simulink model "baleka2S_simscape_frame"  (R2024b)
settings: Solver=VariableStepAuto  StartTime=0.0  StopTime=7.5  RelTol=1e-3
InitFcn:
  | VLcmdsignal = struct( ...
  |     'r_des', 0.45, ...
  |     'dr_des', 0, ...
  |     'th_des', -pi/2, ...
  |     'dth_des', 0, ...
  |     'KPr', 200, ...
  |     'KDr', 2, ...
  |     'KPth', 30, ...
  |     'KDth', 4, ...
  |     'Fff', 0, ...
  |     'Tff', 0);
  | 
  | % run("roll_body_DataFile.m");
  | % run("diff_body_DataFile.m");
undefined symbols (not defined in the file): Kd, Kp, q, tff, w, X, Y, Z
libraries: sm_lib x123, nesl_utility x13, aru_toolbox x11
(part 1 of 3)
settings Model: DataDictionary=Library_dictionary.sldd  Creator=claro  LastModifiedBy=claro

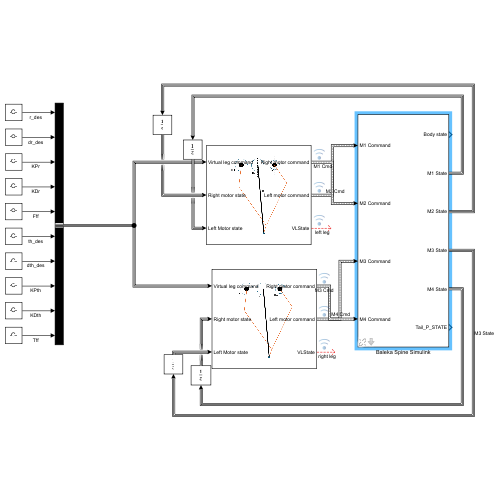
[thumbnail: Simulink's stored preview of the top-level diagram]
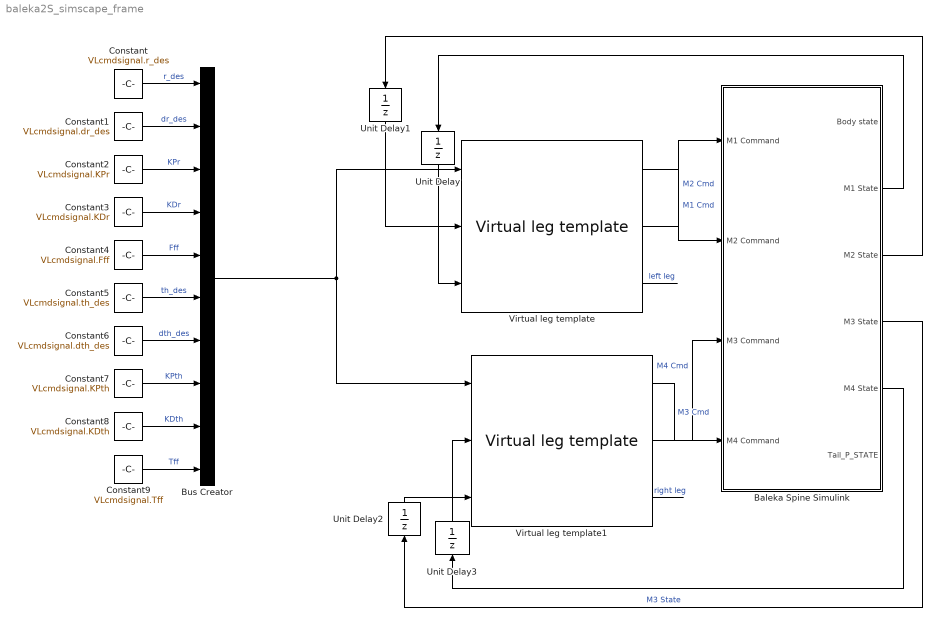
== system baleka2S_simscape_frame ==
  Baleka Spine Simulink : Subsystem  AncestorBlock=aru_toolbox/Baleka 2.5/Baleka Simscape  mask(Simulation model){communication_rate=1000, GravityBool=on, mu_s=1, mu_k=0.9, foot_k=1e5, foot_d=1e4, y_start=0.35, StartingMode=Zero (set Starting values manually), LOffset=2*pi-2.7, ROffset=-0.3}
      mask prompts: communication_rate "Communication Rate"; GravityBool "Enable gravity"; mu_s "Static friction coefficient"; mu_k "Kinetic Friction coefficient"; foot_k "Contact spring constant"; foot_d "Contact damping"; y_start "Boom height (m)"; StartingMode "Starting angle preset"; LOffset "Left motor starting angles (rad)"; ROffset "Right motor starting angles (rad)"
      mask help: The (hopefully) all-in-one model for simulating Baleka 2.5 using Simscape. This model assumes counter clockwise positive, and has busses for both inputs and outputs.
      mask init:
      | if StartingMode == "Crouched"
      |         LmotorOffset = pi-37.63*pi/180; % Measured from Solidworks model and confirmed in Simscape
      |         RmotorOffset = 38.24*pi/180;
      |         LinkStartingRad=1;
      |         
      |     end
      |     if StartingMode == "Links horizontal"
      |         LmotorOffset = pi;
      |         RmotorOffset =0;
      |         LinkStartingRad = 2;
      |     end
      |     if StartingMode == "Zero (set Starting values manually)"
      |         LmotorOffset = LOffset;
      |         RmotorOffset = ROffset;
      |         LinkStartingRad=0;
      |     end
      |    if GravityBool
      |        g = -9.80665;
      |    else
      |        g = 0;
      |    end
      |    th_boom = asin((y_start -0.101)/2.493);
      mask TypeOptions StartingMode: Crouched | Links horizontal | Zero (set Starting values manually)
      mask DialogControl Container3 Prompt: Contacts
      mask DialogControl Container4 Prompt: Starting values
      mask DialogControl Container5 Prompt: Leg angles
      mask DialogControl Control2 Prompt: Custom angles only implimented if starting preset is zero
  Bus Creator : BusCreator  Inputs=10  OutDataTypeStr=Bus: VLcmd
  Constant : Constant  Value=VLcmdsignal.r_des
  Constant1 : Constant  Value=VLcmdsignal.dr_des
  Constant2 : Constant  Value=VLcmdsignal.KPr
  Constant3 : Constant  Value=VLcmdsignal.KDr
  Constant4 : Constant  Value=VLcmdsignal.Fff
  Constant5 : Constant  Value=VLcmdsignal.th_des
  Constant6 : Constant  Value=VLcmdsignal.dth_des
  Constant7 : Constant  Value=VLcmdsignal.KPth
  Constant8 : Constant  Value=VLcmdsignal.KDth
  Constant9 : Constant  Value=VLcmdsignal.Tff
  Unit Delay{,1..3} (4 alike) : UnitDelay  SampleTime=-1  HasFrameUpgradeWarning=on
  Virtual leg template : aru_toolbox/Baleka 2.5/Virtual leg template  SystemSampleTime=-1  VariantActivationTime=update diagram  AllowFlexibleInterface=on  Latency=0  AutoFrameSizeCalculation=off
      settings: SourceProductName=ARU Toolbox
  Virtual leg template1 : aru_toolbox/Baleka 2.5/Virtual leg template  SystemSampleTime=-1  VariantActivationTime=update diagram  AllowFlexibleInterface=on  Latency=0  AutoFrameSizeCalculation=off
      settings: SourceProductName=ARU Toolbox
  wires:
  Virtual leg template/2 -> Baleka Spine Simulink/1(M1 Command)  "M2 Cmd"
  Virtual leg template/1 -> Baleka Spine Simulink/2(M2 Command)  "M1 Cmd"
  Virtual leg template1/1 -> Baleka Spine Simulink/4(M4 Command)  "M3 Cmd"
  Virtual leg template1/2 -> Baleka Spine Simulink/3(M3 Command)  "M4 Cmd"
  Baleka Spine Simulink/4(M3 State) -> Unit Delay2/1  "M3 State"
  Bus Creator/1 -> Virtual leg template/1, Virtual leg template1/1
  Constant/1 -> Bus Creator/1  "r_des"
  Constant1/1 -> Bus Creator/2  "dr_des"
  Constant2/1 -> Bus Creator/3  "KPr"
  Constant3/1 -> Bus Creator/4  "KDr"
  Constant4/1 -> Bus Creator/5  "Fff"
  Constant5/1 -> Bus Creator/6  "th_des"
  Constant6/1 -> Bus Creator/7  "dth_des"
  Constant7/1 -> Bus Creator/8  "KPth"
  Constant8/1 -> Bus Creator/9  "KDth"
  Constant9/1 -> Bus Creator/10  "Tff"
  Unit Delay/1 -> Virtual leg template/3
  Unit Delay1/1 -> Virtual leg template/2
  Unit Delay2/1 -> Virtual leg template1/3
  Unit Delay3/1 -> Virtual leg template1/2
  Baleka Spine Simulink/5(M4 State) -> Unit Delay3/1
  Baleka Spine Simulink/2(M1 State) -> Unit Delay/1
  Baleka Spine Simulink/3(M2 State) -> Unit Delay1/1
  Virtual leg template1/3 -> ?  "right leg"
  Virtual leg template/3 -> ?  "left leg"

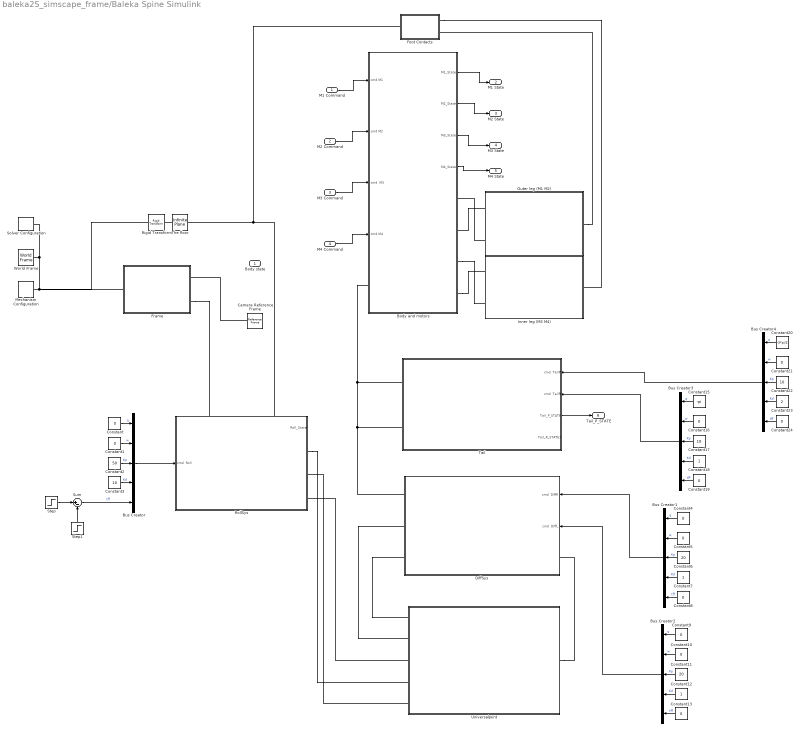
== system baleka2S_simscape_frame/Baleka Spine Simulink ==
  M1 Command : Inport  OutDataTypeStr=Bus: MotorCmd
  M2 Command : Inport  Port=2  OutDataTypeStr=Bus: MotorCmd
  M3 Command : Inport  Port=3  OutDataTypeStr=Bus: MotorCmd
  M4 Command : Inport  Port=4  OutDataTypeStr=Bus: MotorCmd
  " Outer leg (M1 M2)" : Subsystem
  Body and motors : Subsystem
  Bus Creator{,1..4} (5 alike) : BusCreator  Inputs=q,w,Kp,Kd,tff  OutDataTypeStr=Bus: MotorCmd
  Camera Reference Frame : sm_lib/Frames and Transforms/Reference Frame
  Constant{,1,4..5,8..10,13,16,19,21,24} (12 alike) : Constant  Value=0
  Constant11 : Constant  Value=20
  Constant12 : Constant
  Constant15 : Constant  Value=-pi
  Constant17 : Constant  Value=10
  Constant18 : Constant
  Constant2 : Constant  Value=50
  Constant20 : Constant  Value=-3*pi/2
  Constant22 : Constant  Value=10
  Constant23 : Constant  Value=2
  Constant3 : Constant  Value=10
  Constant6 : Constant  Value=20
  Constant7 : Constant
  DiffSys : Subsystem
      settings: PortSchema="{\"entries\":[{\"content\":{\"sides\":[{\"content\":{\"connectorIds\":[\"LConn1\",\"LConn2\",\"LConn3\"]},\"type\":\"ConnectorPlacement.EquallySpacedRectSide\",\"uuid\":\"322efe47-c693-4372-b523-ac4150ea56a3\"},{\"content\":{\"connectorIds\":[\"In1\",\"In2\",\"RConn1\"],\"side\":\"RIGHT\"},\"type\":\"ConnectorPlacement.EquallySpacedRectSide\",\"uuid\":\"9b382245-60e0-481a-af9a-4690adad6086\"},{\"content\":{\"side\":\"TOP\"},\"type\":\"ConnectorPlacement.EquallySpacedRectSide\",\"uuid\":\"0b256e53-2003-47ff-95d4-d002f32bb36d\"},{\"content\":{\"side\":\"BOTTOM\"},\"type\":\"ConnectorPlacement.EquallySpacedRectSide\",\"uuid\":\"ab3905eb-9bc7-48cc-903a-2471c31a1ad7\"}]},\"type\":\"ConnectorPlacement.EquallySpacedConnector\",\"uuid\":\"7ff5e8a9-a8e4-454d-a7ba-3a225b667645\"}],\"packageUris\":[\"http://schema.mathworks.com/mf0/Connector/R2020b\"],\"version\":\"1.0\"}"
  Foot Contacts : Subsystem
  Frame : Subsystem
  Inner leg (M3 M4) : Subsystem
  Mechanism Configuration : sm_lib/Utilities/Mechanism Configuration  UniformGravity=Constant  GravityVector=[0 0 g]  GravityVectorUnits=m/s^2  LinearizationDelta=0.001  JointModeTransitionNonlinearIterations=2
  Rigid Transform : sm_lib/Frames and Transforms/Rigid Transform  RotationMethod=None  FollAlignAxisA=+X  BaseAlignAxisA=+Y  FollAlignAxisB=+Y  BaseAlignAxisB=+Z  RotationStandardAxis=+Z  RotationAngle=0  RotationAngleUnits=deg  RotationArbitraryAxis=[0 0 1]  RotationSequenceAxes=FollowerAxes  RotationSequence=XYX  RotationSequenceAngles=[0 0 0]  RotationSequenceAnglesUnits=deg  RotationMatrix=[1 0 0;0 1 0;0 0 1]  Quaternion=[1 0 0 0]  TranslationMethod=Cartesian  TranslationCartesianOffset=[0 0 4]  TranslationCartesianOffsetUnits=mm  TranslationStandardAxis=+Z  TranslationStandardOffset=0  TranslationStandardOffsetUnits=m  TranslationROffset=0  TranslationROffsetUnits=m  TranslationThetaOffset=0  TranslationThetaOffsetUnits=deg  TranslationZOffset=0  TranslationZOffsetUnits=m
  RollSys : Subsystem
      settings: PortSchema="{\"entries\":[{\"content\":{\"sides\":[{\"content\":{\"connectorIds\":[\"In1\"]},\"type\":\"ConnectorPlacement.EquallySpacedRectSide\",\"uuid\":\"dfefdc23-044e-4fd3-8804-6b125fee8169\"},{\"content\":{\"connectorIds\":[\"Out1\",\"RConn1\",\"RConn2\",\"RConn3\"],\"side\":\"RIGHT\"},\"type\":\"ConnectorPlacement.EquallySpacedRectSide\",\"uuid\":\"fa13e48c-80ad-4683-8483-cd805fea927b\"},{\"content\":{\"connectorIds\":[\"LConn1\",\"LConn2\"],\"side\":\"TOP\"},\"type\":\"ConnectorPlacement.EquallySpacedRectSide\",\"uuid\":\"92ac139b-ee3c-4e16-9e24-f9ffaf9597bb\"}]},\"type\":\"ConnectorPlacement.EquallySpacedConnector\",\"uuid\":\"7d988bd9-98fd-44d8-87f5-37b6f9d1dfc6\"}],\"packageUris\":[\"http://schema.mathworks.com/mf0/Connector/R2020b\"],\"version\":\"1.0\"}"
  Solver Configuration : nesl_utility/Solver Configuration  PhysicalDomain=network_engine_domain  SubClassName=solver  LeftPortType=input  RightPortType=generic  Tones=[]  Harmonics=[]  SimulateNoise=off  Profile=off  UseLocalSampling=off  EnableSwitchedLinearOptims=on  FrequencyDomain=off  UseCCode=off  RelTol=0.001  AbsTol=1e-06  MinStep=1e-09  ToWorkspace=off  RevertToSquareIcSolve=off  NumHomotopyIterations=100  PhasorMode=off  PhasorModeNumHarmonics=1  ConsistencySolver=NEWTON_FTOL  IndexReductionMethod=DerivativeReplacement  DoDC=off  ResidualTolerance=1e-09  ConsistencyTolSource=GLOBAL  ConsistencyAbsTol=0.001  ConsistencyRelTol=0.001  ConsistencyTolFactor=0.001  UseLocalSolver=off  LocalSolverChoice=NE_BACKWARD_EULER_ADVANCER  ResolveIndetEquations=on  FunctionEvalNumThread=1  LocalSolverSampleTime=0.001  DoFixedCost=off  MaxNonlinIter=3  MaxModeIter=2  ComputeImpulses=off  ImpulseIterations=2  LinearAlgebra=Sparse  LinearAlgebraNumThread=0  EquationFormulation=NE_TIME_EF  DelaysMemoryBudget=1024  AutomaticFiltering=on  FilteringTimeConstant=0.001  PartitionStorageMethod=AS_NEEDED  PartitionMemoryBudget=1024  PartitionMethod=FAST  MultibodyUseLocalSolver=off  MultibodyLocalSolverChoice=ODE1  MultibodyLocalSolverSampleTime=0.001
  Step : Step  After=10  SampleTime=0
  Step1 : Step  Time=2  After=10  SampleTime=0
  Sum : Sum  Inputs=|+-
  Tail : Subsystem
      settings: PortSchema="{\"entries\":[{\"content\":{\"sides\":[{\"content\":{\"connectorIds\":[\"LConn1\",\"LConn2\"]},\"type\":\"ConnectorPlacement.EquallySpacedRectSide\",\"uuid\":\"0d9199a2-443f-4f4e-b188-f9e02ae1d5e0\"},{\"content\":{\"connectorIds\":[\"In1\",\"In2\",\"Out1\",\"Out2\"],\"side\":\"RIGHT\"},\"type\":\"ConnectorPlacement.EquallySpacedRectSide\",\"uuid\":\"3ad3a3b8-4ce3-45de-b3b4-6e5c801c1caa\"},{\"content\":{\"side\":\"TOP\"},\"type\":\"ConnectorPlacement.EquallySpacedRectSide\",\"uuid\":\"02569885-0c9e-4662-843f-d7fa07ad01a1\"}]},\"type\":\"ConnectorPlacement.EquallySpacedConnector\",\"uuid\":\"baab52ed-f3e9-4e9c-9101-cd6ccdd98072\"}],\"packageUris\":[\"http://schema.mathworks.com/mf0/Connector/R2020b\"],\"version\":\"1.0\"}"
  The floor : sm_lib/Curves and Surfaces/Infinite Plane  GraphicType=Rectangle  GraphicPlaneWidth=5.8  GraphicPlaneWidthUnits=m  GraphicPlaneHeight=5.8  GraphicPlaneHeightUnits=m  GraphicVisPropType=SimpleVisualProperties  GraphicDiffuseColor=[1 0 0]  GraphicOpacity=0.25  GraphicSpecularColor=[0.5 0.5 0.5 1.0]  GraphicAmbientColor=[0.15 0.15 0.15 1.0]  GraphicEmissiveColor=[0.0 0.0 0.0 1.0]  GraphicShininess=75
  UniversalJoint : Subsystem
  World Frame : sm_lib/Frames and Transforms/World Frame
  Body state : Outport  OutDataTypeStr=Bus: BodyState
  M1 State : Outport  Port=2
  M2 State : Outport  Port=3
  M3 State : Outport  Port=4
  M4 State : Outport  Port=5
  Tail_P_STATE : Outport  Port=6
  wires:
  M4 Command/1 -> Body and motors/4(cmd M4)
  M3 Command/1 -> Body and motors/3(cmd  M3)
  M2 Command/1 -> Body and motors/2(cmd M2)
  M1 Command/1 -> Body and motors/1(cmd M1)
  Body and motors/4(M4_State) -> M4 State/1
  Body and motors/3(M3_State) -> M3 State/1
  Body and motors/2(M2_State) -> M2 State/1
  Body and motors/1(M1_State) -> M1 State/1
  ? -> Body state/1  "body state"
  Bus Creator/1 -> RollSys/1(cmd  Roll)
  Constant/1 -> Bus Creator/1  "q"
  Constant2/1 -> Bus Creator/3  "Kp"
  Constant1/1 -> Bus Creator/2  "w"
  Constant3/1 -> Bus Creator/4  "Kd"
  Step/1 -> Sum/1
  Constant5/1 -> Bus Creator1/2  "w"
  Constant6/1 -> Bus Creator1/3  "Kp"
  Constant4/1 -> Bus Creator1/1  "q"
  Constant7/1 -> Bus Creator1/4  "Kd"
  Bus Creator1/1 -> DiffSys/1(cmd  DiffR)
  Constant8/1 -> Bus Creator1/5  "tff"
  Step1/1 -> Sum/2
  Constant12/1 -> Bus Creator2/4  "Kd"
  Constant9/1 -> Bus Creator2/1  "q"
  Constant11/1 -> Bus Creator2/3  "Kp"
  Constant10/1 -> Bus Creator2/2  "w"
  Constant13/1 -> Bus Creator2/5  "tff"
  Bus Creator2/1 -> DiffSys/2(cmd  DiffL)
  Sum/1 -> Bus Creator/5  "tff"
  Constant21/1 -> Bus Creator4/2  "w"
  Constant19/1 -> Bus Creator3/5  "tff"
  Constant18/1 -> Bus Creator3/4  "Kd"
  Constant16/1 -> Bus Creator3/2  "w"
  Constant17/1 -> Bus Creator3/3  "Kp"
  Bus Creator4/1 -> Tail/1(cmd  TailP)
  Constant22/1 -> Bus Creator4/3  "Kp"
  Constant23/1 -> Bus Creator4/4  "Kd"
  Constant24/1 -> Bus Creator4/5  "tff"
  Tail/1(Tail_P_STATE) -> Tail_P_STATE/1
  Constant15/1 -> Bus Creator3/1  "q"
  Constant20/1 -> Bus Creator4/1  "q"
  Bus Creator3/1 -> Tail/2(cmd  TailR)
  connections:
  The floor/LConn1 -- Rigid Transform/RConn1
  " Outer leg (M1 M2)"/RConn1 -- Foot Contacts/RConn2
  Foot Contacts/RConn1 -- Inner leg (M3 M4)/RConn1
  Body and motors/RConn3 -- Inner leg (M3 M4)/LConn2
  Body and motors/RConn4 -- Inner leg (M3 M4)/LConn1
  " Outer leg (M1 M2)"/LConn2 -- Body and motors/RConn1
  " Outer leg (M1 M2)"/LConn1 -- Body and motors/RConn2
  Foot Contacts/LConn1 -- RollSys/LConn2 -- The floor/RConn1
  DiffSys/LConn1 -- Tail/LConn2 -- Tail/LConn1 -- Body and motors/LConn1
  DiffSys/LConn3 -- UniversalJoint/LConn1
  UniversalJoint/RConn1 -- DiffSys/RConn1
  DiffSys/LConn2 -- UniversalJoint/LConn2
  RollSys/RConn1 -- UniversalJoint/LConn4
  UniversalJoint/LConn5 -- RollSys/RConn2
  UniversalJoint/LConn3 -- RollSys/RConn3
  World Frame/RConn1 -- Frame/LConn1 -- Rigid Transform/LConn1 -- Mechanism Configuration/RConn1 -- Solver Configuration/RConn1
  Camera Reference Frame/RConn1 -- Frame/RConn1
  Frame/RConn2 -- RollSys/LConn1

== system baleka2S_simscape_frame/Baleka Spine Simulink/ Outer leg (M1 M2) ==
  Inner Foot Joint : sm_lib/Joints/Revolute Joint  JointMode=Normal  CompositeWrenchDir=FollowerOnBase  CompositeWrenchFrame=BaseFrame  SenseConstraintForce=off  SenseConstraintTorque=off  SenseTotalForce=off  SenseTotalTorque=off  PositionTargetSpecify=off  PositionTargetPriority=Low  PositionTargetValue=-1  PositionTargetValueUnits=deg  VelocityTargetSpecify=off  VelocityTargetPriority=High  VelocityTargetValue=0  VelocityTargetValueUnits=deg/s  EquilibriumPosition=0  EquilibriumPositionUnits=deg  SpringStiffness=0  SpringStiffnessUnits=N*m/deg  DampingCoefficient=0  DampingCoefficientUnits=N*m/(deg/s)  LowerLimitSpecify=off  LowerLimitBound=0  LowerLimitBoundUnits=deg  LowerLimitStiffness=1e4  LowerLimitStiffnessUnits=N*m/deg  LowerLimitDamping=10  LowerLimitDampingUnits=N*m/(deg/s)  LowerLimitTransitionRegionWidth=0.1  LowerLimitTransitionRegionWidthUnits=deg  UpperLimitSpecify=off  UpperLimitBound=0  UpperLimitBoundUnits=deg  UpperLimitStiffness=1e4  UpperLimitStiffnessUnits=N*m/deg  UpperLimitDamping=10  UpperLimitDampingUnits=N*m/(deg/s)  UpperLimitTransitionRegionWidth=0.1  UpperLimitTransitionRegionWidthUnits=deg  TorqueActuationMode=NoTorque  MotionActuationMode=ComputedMotion  SensePosition=on  SenseVelocity=off  SenseAcceleration=off  SenseTorqueForce=off  SenseLowerLimitTorqueForce=off  SenseUpperLimitTorqueForce=off
  M1 Leg left : Subsystem
  M1 Set axis : sm_lib/Frames and Transforms/Rigid Transform  RotationMethod=StandardAxis  FollAlignAxisA=+X  BaseAlignAxisA=-Y  FollAlignAxisB=+Y  BaseAlignAxisB=+Y  RotationStandardAxis=+Z  RotationAngle=pi/2  RotationAngleUnits=rad  RotationArbitraryAxis=[0 0 1]  RotationSequenceAxes=FollowerAxes  RotationSequence=XYX  RotationSequenceAngles=[0 0 0]  RotationSequenceAnglesUnits=deg  RotationMatrix=[1 0 0;0 1 0;0 0 1]  Quaternion=[1 0 0 0]  TranslationMethod=None  TranslationCartesianOffset=[0 0 0]  TranslationCartesianOffsetUnits=m  TranslationStandardAxis=+Z  TranslationStandardOffset=0  TranslationStandardOffsetUnits=m  TranslationROffset=0  TranslationROffsetUnits=m  TranslationThetaOffset=0  TranslationThetaOffsetUnits=deg  TranslationZOffset=0  TranslationZOffsetUnits=m
  M2 Leg right : Subsystem
  M2 Set axis : sm_lib/Frames and Transforms/Rigid Transform  RotationMethod=StandardAxis  FollAlignAxisA=+X  BaseAlignAxisA=-Y  FollAlignAxisB=+Y  BaseAlignAxisB=+Y  RotationStandardAxis=+Z  RotationAngle=pi/2  RotationAngleUnits=rad  RotationArbitraryAxis=[0 0 1]  RotationSequenceAxes=FollowerAxes  RotationSequence=XYX  RotationSequenceAngles=[0 0 0]  RotationSequenceAnglesUnits=deg  RotationMatrix=[1 0 0;0 1 0;0 0 1]  Quaternion=[1 0 0 0]  TranslationMethod=None  TranslationCartesianOffset=[0 0 0]  TranslationCartesianOffsetUnits=m  TranslationStandardAxis=+Z  TranslationStandardOffset=0  TranslationStandardOffsetUnits=m  TranslationROffset=0  TranslationROffsetUnits=m  TranslationThetaOffset=0  TranslationThetaOffsetUnits=deg  TranslationZOffset=0  TranslationZOffsetUnits=m
  M1 Shaft : PMIOPort  Side=Left
  M2 Shaft : PMIOPort  Port=2  Side=Left
  Outer foot : PMIOPort  Port=3  Side=Right
  connections:
  M1 Set axis/RConn1 -- M1 Leg left/LConn1
  M1 Leg left/RConn1 -- Outer foot/RConn1
  M2 Set axis/LConn1 -- M2 Shaft/RConn1
  M1 Set axis/LConn1 -- M1 Shaft/RConn1
  M2 Set axis/RConn1 -- M2 Leg right/LConn1
  M1 Leg left/RConn2 -- Inner Foot Joint/LConn1
  Inner Foot Joint/RConn1 -- M2 Leg right/RConn1

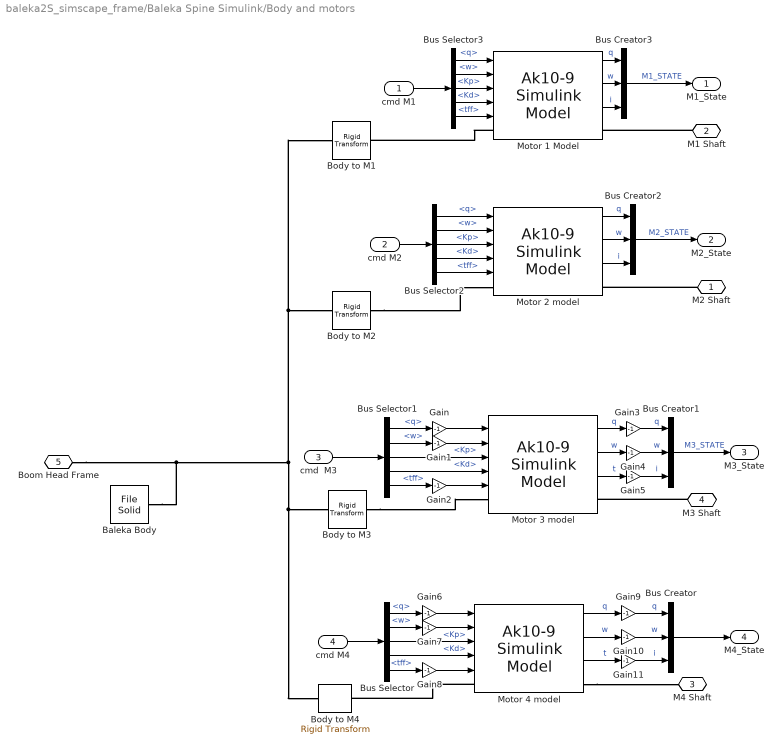
== system baleka2S_simscape_frame/Baleka Spine Simulink/Body and motors ==
  cmd M1 : Inport
  cmd M2 : Inport  Port=2
  cmd  M3 : Inport  Port=3
  cmd M4 : Inport  Port=4
  Baleka Body : sm_lib/Body Elements/File Solid  ExtGeomFileName=simulink-toolbox/Baleka/Meshes/Baleka2_5.STEP  UnitType=Custom  ExtGeomFileUnits=mm  StepReaderType=HEX  ExportConvexHullGeometry=off  InertiaType=Custom  BasedOnType=DensityFromFile  Density=1000  DensityUnits=kg/m^3  Mass=5508.15  MassUnits=g  CenterOfMass=[0.00 6.81 85.00]  CenterOfMassUnits=mm  MomentsOfInertia="[21379023.77  41460427.32 32174580.52]"  MomentsOfInertiaUnits=g*mm^2  ProductsOfInertia=[-0.17, 725.09, -0.35]  ProductsOfInertiaUnits=g*mm^2  GraphicType=FromGeometry  MarkerShape=Sphere  MarkerSize=10  GraphicVisPropType=SimpleVisualProperties  GraphicDiffuseColor=[1.0 1.0 1.0]  GraphicOpacity=0.5  GraphicSpecularColor=[0.5 0.5 0.5 1.0]  GraphicAmbientColor=[0.15 0.15 0.15 1.0]  GraphicEmissiveColor=[0.0 0.0 0.0 1.0]  GraphicShininess=75  DoExposeReferenceFrame=on  SerializedFrames=<Frames/>
  Body to M1 : sm_lib/Frames and Transforms/Rigid Transform  RotationMethod=None  FollAlignAxisA=-X  BaseAlignAxisA=+X  FollAlignAxisB=-Y  BaseAlignAxisB=+Y  RotationStandardAxis=+Z  RotationAngle=0.0  RotationAngleUnits=deg  RotationArbitraryAxis=[0 0 1]  RotationSequenceAxes=FollowerAxes  RotationSequence=XYX  RotationSequenceAngles=[0 0 0]  RotationSequenceAnglesUnits=deg  RotationMatrix=[1 0 0; 0 1 0; 0 0 1]  Quaternion=[1 0 0 0]  TranslationMethod=Cartesian  TranslationCartesianOffset=[-60 0 170]  TranslationCartesianOffsetUnits=mm  TranslationStandardAxis=-X  TranslationStandardOffset=60  TranslationStandardOffsetUnits=mm  TranslationROffset=0  TranslationROffsetUnits=m  TranslationThetaOffset=0  TranslationThetaOffsetUnits=deg  TranslationZOffset=0  TranslationZOffsetUnits=m
  Body to M2 : sm_lib/Frames and Transforms/Rigid Transform  RotationMethod=None  FollAlignAxisA=+X  BaseAlignAxisA=+X  FollAlignAxisB=+Y  BaseAlignAxisB=-Y  RotationStandardAxis=+Z  RotationAngle=0.0  RotationAngleUnits=deg  RotationArbitraryAxis=[0 0 1]  RotationSequenceAxes=FollowerAxes  RotationSequence=XYX  RotationSequenceAngles=[0 0 0]  RotationSequenceAnglesUnits=deg  RotationMatrix=[1 0 0; 0 1 0; 0 0 1]  Quaternion=[1 0 0 0]  TranslationMethod=Cartesian  TranslationCartesianOffset=[60 0 170]  TranslationCartesianOffsetUnits=mm  TranslationStandardAxis=+X  TranslationStandardOffset=60  TranslationStandardOffsetUnits=mm  TranslationROffset=0  TranslationROffsetUnits=m  TranslationThetaOffset=0  TranslationThetaOffsetUnits=deg  TranslationZOffset=0  TranslationZOffsetUnits=m
  Body to M3 : sm_lib/Frames and Transforms/Rigid Transform  RotationMethod=AlignedAxes  FollAlignAxisA=-X  BaseAlignAxisA=+X  FollAlignAxisB=+Z  BaseAlignAxisB=-Z  RotationStandardAxis=+Z  RotationAngle=0.0  RotationAngleUnits=deg  RotationArbitraryAxis=[0 0 1]  RotationSequenceAxes=FollowerAxes  RotationSequence=XYX  RotationSequenceAngles=[0 0 0]  RotationSequenceAnglesUnits=deg  RotationMatrix=[1 0 0; 0 1 0; 0 0 1]  Quaternion=[1 0 0 0]  TranslationMethod=StandardAxis  TranslationCartesianOffset=[0 0 0]  TranslationCartesianOffsetUnits=mm  TranslationStandardAxis=-X  TranslationStandardOffset=60  TranslationStandardOffsetUnits=mm  TranslationROffset=0  TranslationROffsetUnits=m  TranslationThetaOffset=0  TranslationThetaOffsetUnits=deg  TranslationZOffset=0  TranslationZOffsetUnits=m
  Body to M4 : sm_lib/Frames and Transforms/Rigid Transform  RotationMethod=AlignedAxes  FollAlignAxisA=-X  BaseAlignAxisA=+X  FollAlignAxisB=+Z  BaseAlignAxisB=-Z  RotationStandardAxis=+Z  RotationAngle=0.0  RotationAngleUnits=deg  RotationArbitraryAxis=[0 0 1]  RotationSequenceAxes=FollowerAxes  RotationSequence=XYX  RotationSequenceAngles=[0 0 0]  RotationSequenceAnglesUnits=deg  RotationMatrix=[1 0 0; 0 1 0; 0 0 1]  Quaternion=[1 0 0 0]  TranslationMethod=StandardAxis  TranslationCartesianOffset=[0 0 0]  TranslationCartesianOffsetUnits=mm  TranslationStandardAxis=+X  TranslationStandardOffset=60  TranslationStandardOffsetUnits=mm  TranslationROffset=0  TranslationROffsetUnits=m  TranslationThetaOffset=0  TranslationThetaOffsetUnits=deg  TranslationZOffset=0  TranslationZOffsetUnits=m
  Bus Creator{,1..3} (4 alike) : BusCreator  Inputs=3  OutDataTypeStr=Bus: MotorState
  Bus Selector{,1..3} (4 alike) : BusSelector  OutputSignals=q,w,Kp,Kd,tff
  Gain{,1..11} (12 alike) : Gain  Gain=-1
  Motor 1 Model : aru_toolbox/Baleka 2.5/Ak10-9 Simulink Model  J=0.0145  b=0.011  Bt=0.2  Ct=0.1  zero_origin=0  communication_rate=1000  Hip_q0=LmotorOffset  Hip_w0=0
      settings: SourceProductName=ARU Toolbox
  Motor 2 model : aru_toolbox/Baleka 2.5/Ak10-9 Simulink Model  J=0.0145  b=0.011  Bt=0.2  Ct=0.1  zero_origin=0  communication_rate=1000  Hip_q0=RmotorOffset  Hip_w0=0
      settings: SourceProductName=ARU Toolbox
  Motor 3 model : aru_toolbox/Baleka 2.5/Ak10-9 Simulink Model  J=0.0145  b=0.011  Bt=0.2  Ct=0.1  zero_origin=0  communication_rate=1000  Hip_q0=-LmotorOffset  Hip_w0=0
      settings: SourceProductName=ARU Toolbox
  Motor 4 model : aru_toolbox/Baleka 2.5/Ak10-9 Simulink Model  J=0.0145  b=0.011  Bt=0.2  Ct=0.1  zero_origin=0  communication_rate=1000  Hip_q0=-RmotorOffset  Hip_w0=0
      settings: SourceProductName=ARU Toolbox
  M2 Shaft : PMIOPort  Side=Right
  M1 Shaft : PMIOPort  Port=2  Side=Right
  M4 Shaft : PMIOPort  Port=3  Side=Right
  M3 Shaft : PMIOPort  Port=4  Side=Right
  Boom Head Frame : PMIOPort  Port=5  Side=Left
  M1_State : Outport
  M2_State : Outport  Port=2
  M3_State : Outport  Port=3
  M4_State : Outport  Port=4
  wires:
  Gain11/1 -> Bus Creator/3  "i"
  Motor 4 model/3 -> Gain11/1  "t"
  Gain10/1 -> Bus Creator/2  "w"
  Motor 4 model/2 -> Gain10/1  "w"
  Motor 4 model/1 -> Gain9/1  "q"
  Gain9/1 -> Bus Creator/1  "q"
  Gain8/1 -> Motor 4 model/5
  Bus Selector/5 -> Gain8/1  "<tff>"
  Gain7/1 -> Motor 4 model/2
  Bus Selector/2 -> Gain7/1  "<w>"
  Gain6/1 -> Motor 4 model/1
  Bus Selector/1 -> Gain6/1  "<q>"
  Gain5/1 -> Bus Creator1/3  "i"
  Motor 3 model/3 -> Gain5/1  "t"
  Gain4/1 -> Bus Creator1/2  "w"
  Motor 3 model/2 -> Gain4/1  "w"
  Gain3/1 -> Bus Creator1/1  "q"
  Motor 3 model/1 -> Gain3/1  "q"
  Gain2/1 -> Motor 3 model/5
  Bus Selector1/5 -> Gain2/1  "<tff>"
  Gain1/1 -> Motor 3 model/2
  Bus Selector1/2 -> Gain1/1  "<w>"
  Gain/1 -> Motor 3 model/1
  Bus Selector3/5 -> Motor 1 Model/5  "<tff>"
  Bus Creator3/1 -> M1_State/1  "M1_STATE"
  cmd M1/1 -> Bus Selector3/1
  Motor 1 Model/1 -> Bus Creator3/1  "q"
  Motor 1 Model/2 -> Bus Creator3/2  "w"
  Motor 1 Model/3 -> Bus Creator3/3  "i"
  Bus Selector3/4 -> Motor 1 Model/4  "<Kd>"
  Bus Selector3/3 -> Motor 1 Model/3  "<Kp>"
  Bus Selector3/2 -> Motor 1 Model/2  "<w>"
  Bus Selector3/1 -> Motor 1 Model/1  "<q>"
  Bus Creator2/1 -> M2_State/1  "M2_STATE"
  Motor 2 model/2 -> Bus Creator2/2  "w"
  Bus Selector2/4 -> Motor 2 model/4  "<Kd>"
  Motor 2 model/1 -> Bus Creator2/1  "q"
  Bus Selector2/2 -> Motor 2 model/2  "<w>"
  Bus Selector2/5 -> Motor 2 model/5  "<tff>"
  Bus Selector2/1 -> Motor 2 model/1  "<q>"
  Motor 2 model/3 -> Bus Creator2/3  "i"
  Bus Selector2/3 -> Motor 2 model/3  "<Kp>"
  cmd  M3/1 -> Bus Selector1/1
  Bus Selector1/3 -> Motor 3 model/3  "<Kp>"
  Bus Selector1/1 -> Gain/1  "<q>"
  Bus Selector1/4 -> Motor 3 model/4  "<Kd>"
  Bus Creator/1 -> M4_State/1
  Bus Selector/3 -> Motor 4 model/3  "<Kp>"
  Bus Selector/4 -> Motor 4 model/4  "<Kd>"
  cmd M4/1 -> Bus Selector/1
  cmd M2/1 -> Bus Selector2/1
  Bus Creator1/1 -> M3_State/1  "M3_STATE"
  connections:
  M3 Shaft/RConn1 -- Motor 3 model/RConn1
  Motor 4 model/RConn1 -- M4 Shaft/RConn1
  M2 Shaft/RConn1 -- Motor 2 model/RConn1
  M1 Shaft/RConn1 -- Motor 1 Model/RConn1
  Body to M2/RConn1 -- Motor 2 model/LConn1
  Baleka Body/RConn1 -- Body to M3/LConn1 -- Body to M4/LConn1 -- Body to M2/LConn1 -- Body to M1/LConn1 -- Boom Head Frame/RConn1
  Body to M3/RConn1 -- Motor 3 model/LConn1
  Motor 1 Model/LConn1 -- Body to M1/RConn1
  Motor 4 model/LConn1 -- Body to M4/RConn1

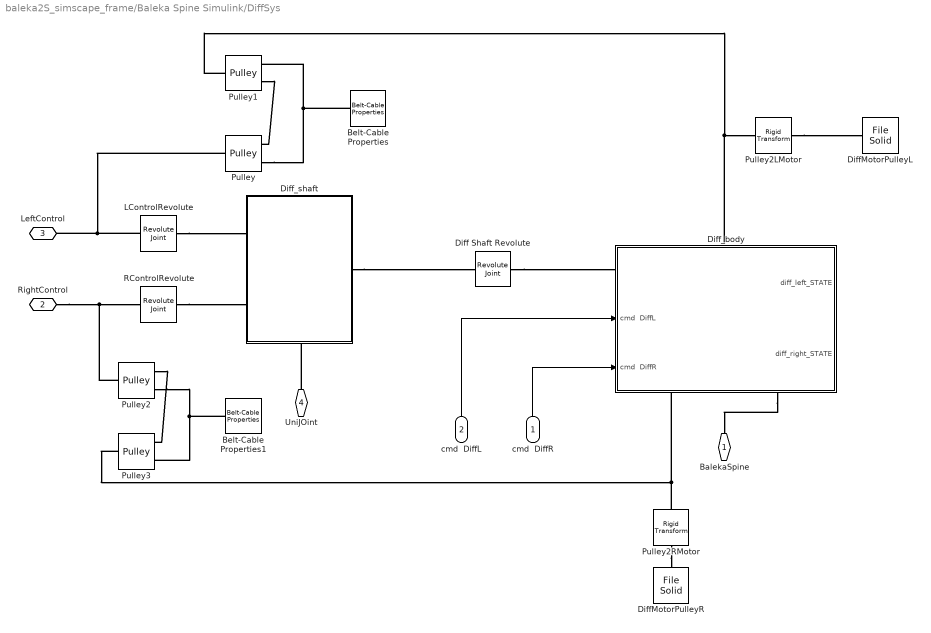
== system baleka2S_simscape_frame/Baleka Spine Simulink/DiffSys ==
  cmd  DiffR : Inport
  cmd  DiffL : Inport  Port=2
  Belt-Cable Properties : sm_lib/Belts and Cables/Belt-Cable Properties  DrumBeltCableAlignment=Unrestricted  GraphicType=PitchLine  GraphicVisPropType=SimpleVisualProperties  GraphicDiffuseColor=[0.5 0.5 0.5]  GraphicOpacity=1  GraphicSpecularColor=[0.5 0.5 0.5 1.0]  GraphicAmbientColor=[0.15 0.15 0.15 1.0]  GraphicEmissiveColor=[0.0 0.0 0.0 1.0]  GraphicShininess=75
  Belt-Cable Properties1 : sm_lib/Belts and Cables/Belt-Cable Properties  DrumBeltCableAlignment=Unrestricted  GraphicType=PitchLine  GraphicVisPropType=SimpleVisualProperties  GraphicDiffuseColor=[0.5 0.5 0.5]  GraphicOpacity=1  GraphicSpecularColor=[0.5 0.5 0.5 1.0]  GraphicAmbientColor=[0.15 0.15 0.15 1.0]  GraphicEmissiveColor=[0.0 0.0 0.0 1.0]  GraphicShininess=75
  Diff Shaft Revolute : sm_lib/Joints/Revolute Joint  JointMode=Normal  CompositeWrenchDir=FollowerOnBase  CompositeWrenchFrame=BaseFrame  SenseConstraintForce=off  SenseConstraintTorque=off  SenseTotalForce=off  SenseTotalTorque=off  PositionTargetSpecify=off  PositionTargetPriority=High  PositionTargetValue=0  PositionTargetValueUnits=deg  VelocityTargetSpecify=off  VelocityTargetPriority=High  VelocityTargetValue=0  VelocityTargetValueUnits=deg/s  EquilibriumPosition=0  EquilibriumPositionUnits=deg  SpringStiffness=0  SpringStiffnessUnits=N*m/deg  DampingCoefficient=0  DampingCoefficientUnits=N*m/(deg/s)  LowerLimitSpecify=off  LowerLimitBound=-90  LowerLimitBoundUnits=deg  LowerLimitStiffness=1e4  LowerLimitStiffnessUnits=N*m/deg  LowerLimitDamping=10  LowerLimitDampingUnits=N*m/(deg/s)  LowerLimitTransitionRegionWidth=0.1  LowerLimitTransitionRegionWidthUnits=deg  UpperLimitSpecify=off  UpperLimitBound=90  UpperLimitBoundUnits=deg  UpperLimitStiffness=1e4  UpperLimitStiffnessUnits=N*m/deg  UpperLimitDamping=10  UpperLimitDampingUnits=N*m/(deg/s)  UpperLimitTransitionRegionWidth=0.1  UpperLimitTransitionRegionWidthUnits=deg  TorqueActuationMode=NoTorque  MotionActuationMode=ComputedMotion  SensePosition=off  SenseVelocity=off  SenseAcceleration=off  SenseTorqueForce=off  SenseLowerLimitTorqueForce=off  SenseUpperLimitTorqueForce=off
  DiffMotorPulleyL : sm_lib/Body Elements/File Solid  ExtGeomFileName=C:\Users\claro\OneDrive - University of Cape Town\BalekaSpine\BalekaSpineMatlab\meshes\PT-48T-5M-15W-12B (Diff motor).STEP  UnitType=Custom  ExtGeomFileUnits=mm  StepReaderType=HEX  ExportConvexHullGeometry=off  InertiaType=Custom  BasedOnType=DensityFromFile  Density=1000  DensityUnits=kg/m^3  Mass=0.08598  MassUnits=kg  CenterOfMass=[0.00000, 0.00854, 0.00000]  CenterOfMassUnits=m  MomentsOfInertia=[3.26079400e-05, 5.80122000e-05, 3.26079400e-05]  MomentsOfInertiaUnits=kg*m^2  ProductsOfInertia=[0.00000000e+00, 0.00000000e+00, 0.00000000e+00]  ProductsOfInertiaUnits=kg*m^2  GraphicType=FromGeometry  MarkerShape=Sphere  MarkerSize=10  GraphicVisPropType=SimpleVisualProperties  GraphicDiffuseColor=[0.5 0.5 0.5]  GraphicOpacity=1  GraphicSpecularColor=[0.5 0.5 0.5 1.0]  GraphicAmbientColor=[0.15 0.15 0.15 1.0]  GraphicEmissiveColor=[0.0 0.0 0.0 1.0]  GraphicShininess=75  DoExposeReferenceFrame=on  SerializedFrames=<Frames/>
  DiffMotorPulleyR : sm_lib/Body Elements/File Solid  ExtGeomFileName=C:\Users\claro\OneDrive - University of Cape Town\BalekaSpine\BalekaSpineMatlab\meshes\PT-48T-5M-15W-12B (Diff motor).STEP  UnitType=Custom  ExtGeomFileUnits=mm  StepReaderType=HEX  ExportConvexHullGeometry=off  InertiaType=Custom  BasedOnType=DensityFromFile  Density=1000  DensityUnits=kg/m^3  Mass=0.08598  MassUnits=kg  CenterOfMass=[0.00000, 0.00854, 0.00000]  CenterOfMassUnits=m  MomentsOfInertia=[3.26079400e-05, 5.80122000e-05, 3.26079400e-05]  MomentsOfInertiaUnits=kg*m^2  ProductsOfInertia=[0.00000000e+00, 0.00000000e+00, 0.00000000e+00]  ProductsOfInertiaUnits=kg*m^2  GraphicType=FromGeometry  MarkerShape=Sphere  MarkerSize=10  GraphicVisPropType=SimpleVisualProperties  GraphicDiffuseColor=[0.5 0.5 0.5]  GraphicOpacity=1  GraphicSpecularColor=[0.5 0.5 0.5 1.0]  GraphicAmbientColor=[0.15 0.15 0.15 1.0]  GraphicEmissiveColor=[0.0 0.0 0.0 1.0]  GraphicShininess=75  DoExposeReferenceFrame=on  SerializedFrames=<Frames/>
  Diff_body : Subsystem
      settings: PortSchema="{\"entries\":[{\"content\":{\"sides\":[{\"content\":{\"connectorIds\":[\"LConn1\",\"In1\",\"In2\"]},\"type\":\"ConnectorPlacement.EquallySpacedRectSide\",\"uuid\":\"ca795cbb-773b-4b56-9b99-04547e78aa1d\"},{\"content\":{\"connectorIds\":[\"Out1\",\"Out2\"],\"side\":\"RIGHT\"},\"type\":\"ConnectorPlacement.EquallySpacedRectSide\",\"uuid\":\"8954f6d9-4de6-40c8-8ccf-9041b0054f85\"},{\"content\":{\"connectorIds\":[\"LConn2\"],\"side\":\"TOP\"},\"type\":\"ConnectorPlacement.EquallySpacedRectSide\",\"uuid\":\"074fe64f-9ff5-4700-85db-ab2eae463c73\"},{\"content\":{\"connectorIds\":[\"RConn1\",\"RConn2\"],\"side\":\"BOTTOM\"},\"type\":\"ConnectorPlacement.EquallySpacedRectSide\",\"uuid\":\"efaddfc6-2460-4fe4-94c5-7333f5a200bc\"}]},\"type\":\"ConnectorPlacement.EquallySpacedConnector\",\"uuid\":\"f94cef8e-b549-4da6-9cca-df567dd62534\"}],\"packageUris\":[\"http://schema.mathworks.com/mf0/Connector/R2020b\"],\"version\":\"1.0\"}"
  Diff_shaft : Subsystem
      settings: PortSchema="{\"entries\":[{\"content\":{\"sides\":[{\"content\":{\"connectorIds\":[\"LConn1\",\"LConn2\"]},\"type\":\"ConnectorPlacement.EquallySpacedRectSide\",\"uuid\":\"37f827ce-2b7c-4f9f-804e-85f40b9d63a7\"},{\"content\":{\"connectorIds\":[\"RConn1\"],\"side\":\"RIGHT\"},\"type\":\"ConnectorPlacement.EquallySpacedRectSide\",\"uuid\":\"b631bcf8-ce7e-4874-ab4d-685d90dbbdf3\"},{\"content\":{\"side\":\"TOP\"},\"type\":\"ConnectorPlacement.EquallySpacedRectSide\",\"uuid\":\"a406f9dd-1146-44b4-821f-545d9f0c91a5\"},{\"content\":{\"connectorIds\":[\"RConn2\"],\"side\":\"BOTTOM\"},\"type\":\"ConnectorPlacement.EquallySpacedRectSide\",\"uuid\":\"20ebd017-15f9-4fad-9c94-d50a3217c3bf\"}]},\"type\":\"ConnectorPlacement.EquallySpacedConnector\",\"uuid\":\"c4dc00e2-1e5d-47f7-b8f1-f0c7deacac21\"}],\"packageUris\":[\"http://schema.mathworks.com/mf0/Connector/R2020b\"],\"version\":\"1.0\"}"
  LControlRevolute : sm_lib/Joints/Revolute Joint  JointMode=Normal  CompositeWrenchDir=FollowerOnBase  CompositeWrenchFrame=BaseFrame  SenseConstraintForce=off  SenseConstraintTorque=off  SenseTotalForce=off  SenseTotalTorque=off  PositionTargetSpecify=off  PositionTargetPriority=High  PositionTargetValue=0  PositionTargetValueUnits=deg  VelocityTargetSpecify=off  VelocityTargetPriority=High  VelocityTargetValue=0  VelocityTargetValueUnits=deg/s  EquilibriumPosition=0  EquilibriumPositionUnits=deg  SpringStiffness=0  SpringStiffnessUnits=N*m/deg  DampingCoefficient=0  DampingCoefficientUnits=N*m/(deg/s)  LowerLimitSpecify=off  LowerLimitBound=-90  LowerLimitBoundUnits=deg  LowerLimitStiffness=1e4  LowerLimitStiffnessUnits=N*m/deg  LowerLimitDamping=10  LowerLimitDampingUnits=N*m/(deg/s)  LowerLimitTransitionRegionWidth=0.1  LowerLimitTransitionRegionWidthUnits=deg  UpperLimitSpecify=off  UpperLimitBound=90  UpperLimitBoundUnits=deg  UpperLimitStiffness=1e4  UpperLimitStiffnessUnits=N*m/deg  UpperLimitDamping=10  UpperLimitDampingUnits=N*m/(deg/s)  UpperLimitTransitionRegionWidth=0.1  UpperLimitTransitionRegionWidthUnits=deg  TorqueActuationMode=NoTorque  MotionActuationMode=ComputedMotion  SensePosition=off  SenseVelocity=off  SenseAcceleration=off  SenseTorqueForce=off  SenseLowerLimitTorqueForce=off  SenseUpperLimitTorqueForce=off
  Pulley{,1..3} (4 alike) : sm_lib/Belts and Cables/Pulley  PitchRadius=76/2  PitchRadiusUnits=mm  InitialWrapAngleLowerBound=0  InitialWrapAngleLowerBoundUnits=deg  SenseWrapAngle=off  SensePulleyAngleA=off  SensePulleyAngleB=off  SenseFleetAngleA=off  SenseFleetAngleB=off
  "Pulley2LMotor " : sm_lib/Frames and Transforms/Rigid Transform  RotationMethod=StandardAxis  FollAlignAxisA=+X  BaseAlignAxisA=+Y  FollAlignAxisB=+Y  BaseAlignAxisB=+Z  RotationStandardAxis=-X  RotationAngle=90  RotationAngleUnits=deg  RotationArbitraryAxis=[0 0 1]  RotationSequenceAxes=FollowerAxes  RotationSequence=ZYX  RotationSequenceAngles=[0 0 -90]  RotationSequenceAnglesUnits=deg  RotationMatrix=[1 0 0;0 1 0;0 0 1]  Quaternion=[1 0 0 0]  TranslationMethod=Cartesian  TranslationCartesianOffset=[0 5 0]  TranslationCartesianOffsetUnits=mm  TranslationStandardAxis=+Z  TranslationStandardOffset=0  TranslationStandardOffsetUnits=m  TranslationROffset=0  TranslationROffsetUnits=m  TranslationThetaOffset=0  TranslationThetaOffsetUnits=deg  TranslationZOffset=0  TranslationZOffsetUnits=m
  Pulley2RMotor : sm_lib/Frames and Transforms/Rigid Transform  RotationMethod=StandardAxis  FollAlignAxisA=+X  BaseAlignAxisA=+Y  FollAlignAxisB=+Y  BaseAlignAxisB=+Z  RotationStandardAxis=-X  RotationAngle=90  RotationAngleUnits=deg  RotationArbitraryAxis=[0 0 1]  RotationSequenceAxes=FollowerAxes  RotationSequence=ZYX  RotationSequenceAngles=[0 0 -90]  RotationSequenceAnglesUnits=deg  RotationMatrix=[1 0 0;0 1 0;0 0 1]  Quaternion=[1 0 0 0]  TranslationMethod=Cartesian  TranslationCartesianOffset=[0 5 0]  TranslationCartesianOffsetUnits=mm  TranslationStandardAxis=+Z  TranslationStandardOffset=0  TranslationStandardOffsetUnits=m  TranslationROffset=0  TranslationROffsetUnits=m  TranslationThetaOffset=0  TranslationThetaOffsetUnits=deg  TranslationZOffset=0  TranslationZOffsetUnits=m
  RControlRevolute : sm_lib/Joints/Revolute Joint  JointMode=Normal  CompositeWrenchDir=FollowerOnBase  CompositeWrenchFrame=BaseFrame  SenseConstraintForce=off  SenseConstraintTorque=off  SenseTotalForce=off  SenseTotalTorque=off  PositionTargetSpecify=off  PositionTargetPriority=High  PositionTargetValue=0  PositionTargetValueUnits=deg  VelocityTargetSpecify=off  VelocityTargetPriority=High  VelocityTargetValue=100  VelocityTargetValueUnits=deg/s  EquilibriumPosition=0  EquilibriumPositionUnits=deg  SpringStiffness=0  SpringStiffnessUnits=N*m/deg  DampingCoefficient=0  DampingCoefficientUnits=N*m/(deg/s)  LowerLimitSpecify=off  LowerLimitBound=-90  LowerLimitBoundUnits=deg  LowerLimitStiffness=1e4  LowerLimitStiffnessUnits=N*m/deg  LowerLimitDamping=10  LowerLimitDampingUnits=N*m/(deg/s)  LowerLimitTransitionRegionWidth=0.1  LowerLimitTransitionRegionWidthUnits=deg  UpperLimitSpecify=off  UpperLimitBound=90  UpperLimitBoundUnits=deg  UpperLimitStiffness=1e4  UpperLimitStiffnessUnits=N*m/deg  UpperLimitDamping=10  UpperLimitDampingUnits=N*m/(deg/s)  UpperLimitTransitionRegionWidth=0.1  UpperLimitTransitionRegionWidthUnits=deg  TorqueActuationMode=NoTorque  MotionActuationMode=ComputedMotion  SensePosition=off  SenseVelocity=off  SenseAcceleration=off  SenseTorqueForce=off  SenseLowerLimitTorqueForce=off  SenseUpperLimitTorqueForce=off
  BalekaSpine : PMIOPort  Side=Left
  RightControl : PMIOPort  Port=2  Side=Left
  LeftControl : PMIOPort  Port=3  Side=Left
  UniJOint : PMIOPort  Port=4  Side=Right
  wires:
  cmd  DiffL/1 -> Diff_body/1(cmd  DiffL)
  cmd  DiffR/1 -> Diff_body/2(cmd  DiffR)
  connections:
  Diff Shaft Revolute/LConn1 -- Diff_body/LConn1
  Diff_shaft/RConn1 -- Diff Shaft Revolute/RConn1
  UniJOint/RConn1 -- Diff_shaft/RConn2
  Diff_body/RConn2 -- BalekaSpine/RConn1
  Pulley2RMotor/LConn1 -- DiffMotorPulleyR/RConn1
  "Pulley2LMotor "/LConn1 -- DiffMotorPulleyL/RConn1
  RControlRevolute/LConn1 -- Diff_shaft/LConn2
  RightControl/RConn1 -- Pulley2/LConn1 -- RControlRevolute/RConn1
  Pulley2RMotor/RConn1 -- Diff_body/RConn1 -- Pulley3/LConn1
  Diff_body/LConn2 -- Pulley1/LConn1 -- "Pulley2LMotor "/RConn1
  LControlRevolute/LConn1 -- Diff_shaft/LConn1
  LControlRevolute/RConn1 -- Pulley/LConn1 -- LeftControl/RConn1
  Pulley1/RConn2 -- Pulley/RConn1
  Pulley/RConn2 -- Belt-Cable Properties/LConn1 -- Pulley1/RConn1
  Pulley2/RConn1 -- Pulley3/RConn1
  Pulley2/RConn2 -- Belt-Cable Properties1/LConn1 -- Pulley3/RConn2

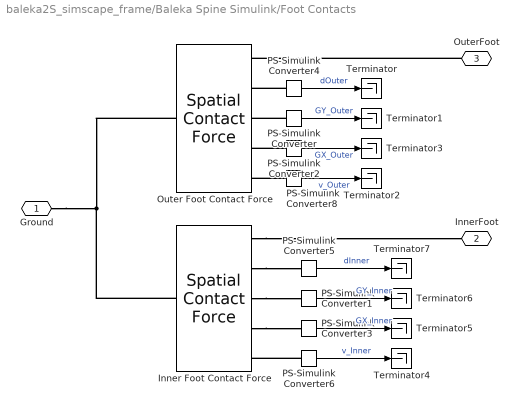
== system baleka2S_simscape_frame/Baleka Spine Simulink/Foot Contacts ==
  Inner Foot Contact Force : sm_lib/Forces and Torques/Spatial Contact Force  NormalForceType=SmoothSpringDamper  NormalStiffness=foot_k  NormalStiffnessUnits=N/m  NormalDamping=foot_d  NormalDampingUnits=N/(m/s)  NormalTransitionRegionWidth=1e-3  NormalTransitionRegionWidthUnits=m  FrictionType=SmoothStickSlip  CoefficientOfStaticFriction=mu_s  CoefficientOfDynamicFriction=mu_k  FrictionalCriticalVelocity=1e-3  FrictionalCriticalVelocityUnits=m/s  SenseContactSignal=off  SensePenetrationDepth=off  SenseSeparationDistance=on  SenseNormalForceMagnitude=on  SenseFrictionalForceMagnitude=on  SenseNormalVelocity=on  SenseTangentialVelocity=off  SenseContactBaseRotation=off  SenseContactBaseTranslation=off  SenseContactFollowerRotation=off  SenseContactFollowerTranslation=off  ZeroCrossDetectContactStartAndEnd=on
  Outer Foot Contact Force : sm_lib/Forces and Torques/Spatial Contact Force  NormalForceType=SmoothSpringDamper  NormalStiffness=foot_k  NormalStiffnessUnits=N/m  NormalDamping=foot_d  NormalDampingUnits=N/(m/s)  NormalTransitionRegionWidth=1e-3  NormalTransitionRegionWidthUnits=m  FrictionType=SmoothStickSlip  CoefficientOfStaticFriction=mu_s  CoefficientOfDynamicFriction=mu_k  FrictionalCriticalVelocity=1e-3  FrictionalCriticalVelocityUnits=m/s  SenseContactSignal=off  SensePenetrationDepth=off  SenseSeparationDistance=on  SenseNormalForceMagnitude=on  SenseFrictionalForceMagnitude=on  SenseNormalVelocity=on  SenseTangentialVelocity=off  SenseContactBaseRotation=off  SenseContactBaseTranslation=off  SenseContactFollowerRotation=off  SenseContactFollowerTranslation=off  ZeroCrossDetectContactStartAndEnd=on
  PS-Simulink Converter{,1..6,8} (8 alike) : nesl_utility/PS-Simulink Converter  PhysicalDomain=network_engine_domain  SubClassName=ps_output  LeftPortType=input  RightPortType=output  PseudoPeriodic=off  Frequencies=[]  VectorFormat=inherit  Unit=inherit  AffineConversion=off
  Terminator{,1..7} (8 alike) : Terminator
  Ground : PMIOPort  Side=Left
  InnerFoot : PMIOPort  Port=2  Side=Right
  OuterFoot : PMIOPort  Port=3  Side=Right
  wires:
  PS-Simulink Converter8/1 -> Terminator2/1  "v_Outer"
  PS-Simulink Converter6/1 -> Terminator4/1  "v_Inner"
  PS-Simulink Converter5/1 -> Terminator7/1  "dInner"
  PS-Simulink Converter1/1 -> Terminator6/1  "GY_Inner"
  PS-Simulink Converter3/1 -> Terminator5/1  "GX_Inner"
  PS-Simulink Converter4/1 -> Terminator/1  "dOuter"
  PS-Simulink Converter2/1 -> Terminator3/1  "GX_Outer"
  PS-Simulink Converter/1 -> Terminator1/1  "GY_Outer"
  connections:
  OuterFoot/RConn1 -- Outer Foot Contact Force/RConn1
  PS-Simulink Converter8/LConn1 -- Outer Foot Contact Force/RConn5
  PS-Simulink Converter6/LConn1 -- Inner Foot Contact Force/RConn5
  Inner Foot Contact Force/RConn4 -- PS-Simulink Converter3/LConn1
  Inner Foot Contact Force/RConn3 -- PS-Simulink Converter1/LConn1
  Inner Foot Contact Force/RConn2 -- PS-Simulink Converter5/LConn1
  PS-Simulink Converter4/LConn1 -- Outer Foot Contact Force/RConn2
  PS-Simulink Converter/LConn1 -- Outer Foot Contact Force/RConn3
  PS-Simulink Converter2/LConn1 -- Outer Foot Contact Force/RConn4
  Inner Foot Contact Force/RConn1 -- InnerFoot/RConn1
  Outer Foot Contact Force/LConn1 -- Inner Foot Contact Force/LConn1 -- Ground/RConn1

== system baleka2S_simscape_frame/Baleka Spine Simulink/Frame ==
  Extrusion Frame : sm_lib/Body Elements/File Solid  ExtGeomFileName=C:\Users\claro\OneDrive - University of Cape Town\BalekaSpine\BalekaSpineMatlab\meshes\baleka_spine_frame_assem.STEP  UnitType=Custom  ExtGeomFileUnits=mm  StepReaderType=HEX  ExportConvexHullGeometry=off  InertiaType=Custom  BasedOnType=DensityFromFile  Density=1000  DensityUnits=kg/m^3  Mass=16.3948  MassUnits=kg  CenterOfMass=[0.00004, 0.01635, 0.0]  CenterOfMassUnits=m  MomentsOfInertia=[202931161.59, 323808867.19, 192898363.67] *1e-9  MomentsOfInertiaUnits=kg*m^2  ProductsOfInertia=[0.0, 0.0, 129751.35] *1e-9  ProductsOfInertiaUnits=kg*m^2  GraphicType=FromGeometry  MarkerShape=Sphere  MarkerSize=10  GraphicVisPropType=SimpleVisualProperties  GraphicDiffuseColor=[0.5 0.5 0.5]  GraphicOpacity=1  GraphicSpecularColor=[0.5 0.5 0.5 1.0]  GraphicAmbientColor=[0.15 0.15 0.15 1.0]  GraphicEmissiveColor=[0.0 0.0 0.0 1.0]  GraphicShininess=75  DoExposeReferenceFrame=on  SerializedFrames=<Frames/>
  Frame Plate : sm_lib/Body Elements/File Solid  ExtGeomFileName=C:\Users\claro\OneDrive - University of Cape Town\BalekaSpine\BalekaSpineMatlab\meshes\BLKS-SM010-roll_plate_frame.STEP  UnitType=Custom  ExtGeomFileUnits=mm  StepReaderType=HEX  ExportConvexHullGeometry=off  InertiaType=Custom  BasedOnType=DensityFromFile  Density=1000  DensityUnits=kg/m^3  Mass=0  MassUnits=kg  CenterOfMass=[0 0 0]  CenterOfMassUnits=m  MomentsOfInertia=[1 1 1]  MomentsOfInertiaUnits=kg*m^2  ProductsOfInertia=[0 0 0]  ProductsOfInertiaUnits=kg*m^2  GraphicType=FromGeometry  MarkerShape=Sphere  MarkerSize=10  GraphicVisPropType=SimpleVisualProperties  GraphicDiffuseColor=[0.5 0.5 0.5]  GraphicOpacity=1  GraphicSpecularColor=[0.5 0.5 0.5 1.0]  GraphicAmbientColor=[0.15 0.15 0.15 1.0]  GraphicEmissiveColor=[0.0 0.0 0.0 1.0]  GraphicShininess=75  DoExposeReferenceFrame=on  SerializedFrames=<Frames/>
  Frame2Plate : sm_lib/Frames and Transforms/Rigid Transform  RotationMethod=RotationSequence  FollAlignAxisA=+X  BaseAlignAxisA=+Y  FollAlignAxisB=+Y  BaseAlignAxisB=+Z  RotationStandardAxis=+X  RotationAngle=90  RotationAngleUnits=deg  RotationArbitraryAxis=[0 0 1]  RotationSequenceAxes=FollowerAxes  RotationSequence=XYZ  RotationSequenceAngles=[90 0 90]  RotationSequenceAnglesUnits=deg  RotationMatrix=[1 0 0;0 1 0;0 0 1]  Quaternion=[1 0 0 0]  TranslationMethod=Cartesian  TranslationCartesianOffset=[16.5 400 0]  TranslationCartesianOffsetUnits=mm  TranslationStandardAxis=+Z  TranslationStandardOffset=0  TranslationStandardOffsetUnits=m  TranslationROffset=0  TranslationROffsetUnits=m  TranslationThetaOffset=0  TranslationThetaOffsetUnits=deg  TranslationZOffset=0  TranslationZOffsetUnits=m
  FramePlate2Roll : sm_lib/Frames and Transforms/Rigid Transform  RotationMethod=RotationSequence  FollAlignAxisA=+X  BaseAlignAxisA=+Y  FollAlignAxisB=+Y  BaseAlignAxisB=+Z  RotationStandardAxis=-X  RotationAngle=270  RotationAngleUnits=deg  RotationArbitraryAxis=[0 0 1]  RotationSequenceAxes=FollowerAxes  RotationSequence=XYZ  RotationSequenceAngles=[-90 180 0]  RotationSequenceAnglesUnits=deg  RotationMatrix=[1 0 0;0 1 0;0 0 1]  Quaternion=[1 0 0 0]  TranslationMethod=Cartesian  TranslationCartesianOffset=[0 133 0]  TranslationCartesianOffsetUnits=mm  TranslationStandardAxis=+Z  TranslationStandardOffset=0  TranslationStandardOffsetUnits=m  TranslationROffset=0  TranslationROffsetUnits=m  TranslationThetaOffset=0  TranslationThetaOffsetUnits=deg  TranslationZOffset=0  TranslationZOffsetUnits=m
  Rigid Transform1 : sm_lib/Frames and Transforms/Rigid Transform  RotationMethod=StandardAxis  FollAlignAxisA=+X  BaseAlignAxisA=+Y  FollAlignAxisB=+Y  BaseAlignAxisB=+Z  RotationStandardAxis=+X  RotationAngle=90  RotationAngleUnits=deg  RotationArbitraryAxis=[0 0 1]  RotationSequenceAxes=FollowerAxes  RotationSequence=XYX  RotationSequenceAngles=[0 0 0]  RotationSequenceAnglesUnits=deg  RotationMatrix=[1 0 0;0 1 0;0 0 1]  Quaternion=[1 0 0 0]  TranslationMethod=None  TranslationCartesianOffset=[0 0 0]  TranslationCartesianOffsetUnits=m  TranslationStandardAxis=+Z  TranslationStandardOffset=0  TranslationStandardOffsetUnits=m  TranslationROffset=0  TranslationROffsetUnits=m  TranslationThetaOffset=0  TranslationThetaOffsetUnits=deg  TranslationZOffset=0  TranslationZOffsetUnits=m
  World : PMIOPort  Side=Left
  Frame : PMIOPort  Port=2  Side=Right
  Roll : PMIOPort  Port=3  Side=Right
  connections:
  Rigid Transform1/RConn1 -- Frame2Plate/LConn1 -- Extrusion Frame/RConn1
  Frame Plate/RConn1 -- Frame/RConn1 -- FramePlate2Roll/LConn1 -- Frame2Plate/RConn1
  FramePlate2Roll/RConn1 -- Roll/RConn1
  World/RConn1 -- Rigid Transform1/LConn1

== system baleka2S_simscape_frame/Baleka Spine Simulink/Inner leg (M3 M4) ==
  Inner foot joint : sm_lib/Joints/Revolute Joint  JointMode=Normal  CompositeWrenchDir=FollowerOnBase  CompositeWrenchFrame=BaseFrame  SenseConstraintForce=off  SenseConstraintTorque=off  SenseTotalForce=off  SenseTotalTorque=off  PositionTargetSpecify=off  PositionTargetPriority=Low  PositionTargetValue=-1  PositionTargetValueUnits=deg  VelocityTargetSpecify=off  VelocityTargetPriority=High  VelocityTargetValue=0  VelocityTargetValueUnits=deg/s  EquilibriumPosition=0  EquilibriumPositionUnits=deg  SpringStiffness=0  SpringStiffnessUnits=N*m/deg  DampingCoefficient=0  DampingCoefficientUnits=N*m/(deg/s)  LowerLimitSpecify=off  LowerLimitBound=0  LowerLimitBoundUnits=deg  LowerLimitStiffness=1e4  LowerLimitStiffnessUnits=N*m/deg  LowerLimitDamping=10  LowerLimitDampingUnits=N*m/(deg/s)  LowerLimitTransitionRegionWidth=0.1  LowerLimitTransitionRegionWidthUnits=deg  UpperLimitSpecify=off  UpperLimitBound=0  UpperLimitBoundUnits=rad  UpperLimitStiffness=1e4  UpperLimitStiffnessUnits=N*m/deg  UpperLimitDamping=10  UpperLimitDampingUnits=N*m/(deg/s)  UpperLimitTransitionRegionWidth=0.1  UpperLimitTransitionRegionWidthUnits=deg  TorqueActuationMode=NoTorque  MotionActuationMode=ComputedMotion  SensePosition=on  SenseVelocity=off  SenseAcceleration=off  SenseTorqueForce=off  SenseLowerLimitTorqueForce=off  SenseUpperLimitTorqueForce=off
  M3 Leg left : Subsystem
  "M3 Set axis " : sm_lib/Frames and Transforms/Rigid Transform  RotationMethod=StandardAxis  FollAlignAxisA=+X  BaseAlignAxisA=-Y  FollAlignAxisB=+Y  BaseAlignAxisB=+Y  RotationStandardAxis=-Z  RotationAngle=pi/2  RotationAngleUnits=rad  RotationArbitraryAxis=[0 0 1]  RotationSequenceAxes=FollowerAxes  RotationSequence=XYX  RotationSequenceAngles=[0 0 0]  RotationSequenceAnglesUnits=deg  RotationMatrix=[1 0 0;0 1 0;0 0 1]  Quaternion=[1 0 0 0]  TranslationMethod=None  TranslationCartesianOffset=[0 0 0]  TranslationCartesianOffsetUnits=m  TranslationStandardAxis=+Z  TranslationStandardOffset=0  TranslationStandardOffsetUnits=m  TranslationROffset=0  TranslationROffsetUnits=m  TranslationThetaOffset=0  TranslationThetaOffsetUnits=deg  TranslationZOffset=0  TranslationZOffsetUnits=m
  M4 Leg right : Subsystem
  M4 Set axis : sm_lib/Frames and Transforms/Rigid Transform  RotationMethod=StandardAxis  FollAlignAxisA=+X  BaseAlignAxisA=-Y  FollAlignAxisB=+Y  BaseAlignAxisB=+Y  RotationStandardAxis=-Z  RotationAngle=pi/2  RotationAngleUnits=rad  RotationArbitraryAxis=[0 0 1]  RotationSequenceAxes=FollowerAxes  RotationSequence=XYX  RotationSequenceAngles=[0 0 0]  RotationSequenceAnglesUnits=deg  RotationMatrix=[1 0 0;0 1 0;0 0 1]  Quaternion=[1 0 0 0]  TranslationMethod=None  TranslationCartesianOffset=[0 0 0]  TranslationCartesianOffsetUnits=m  TranslationStandardAxis=+Z  TranslationStandardOffset=0  TranslationStandardOffsetUnits=m  TranslationROffset=0  TranslationROffsetUnits=m  TranslationThetaOffset=0  TranslationThetaOffsetUnits=deg  TranslationZOffset=0  TranslationZOffsetUnits=m
  M3 Shaft : PMIOPort  Side=Left
  M4 Shaft : PMIOPort  Port=2  Side=Left
  Inner foot : PMIOPort  Port=3  Side=Right
  connections:
  "M3 Set axis "/RConn1 -- M3 Leg left/LConn1
  M3 Leg left/RConn1 -- Inner foot/RConn1
  M4 Set axis/RConn1 -- M4 Leg right/LConn1
  M4 Set axis/LConn1 -- M4 Shaft/RConn1
  "M3 Set axis "/LConn1 -- M3 Shaft/RConn1
  M3 Leg left/RConn2 -- Inner foot joint/LConn1
  M4 Leg right/RConn1 -- Inner foot joint/RConn1
